simulink model "odziv"  (R2020b)
settings: Solver=ode45  StartTime=0.0  StopTime=Tkon  RelTol=1e-3  EnableMultiTasking=on
libraries: PoKeysIOInterface x1
settings Model: Creator=Administrator  LastModifiedBy=Administrator
settings DataIOCC: LimitDataPoints=on  SaveFormat=Array  ReturnWorkspaceOutputs=off
settings OptimizationCC: LifeSpan=inf
settings DebuggingCC: SolverPrmCheckMsg=warning  SFUnexpectedBacktrackingDiag=warning  SFNoUnconditionalDefaultTransitionDiag=warning  SFExecutionAtInitializationDiag=none  ArithmeticOperatorsInVariantConditions=warning
settings HardwareCC: ProdBitPerPointer=32  ProdBitPerSizeT=32  ProdBitPerPtrDiffT=32  ProdLargestAtomicFloat=None  ProdIntDivRoundTo=Undefined  ProdEndianess=Unspecified  ProdWordSize=32  ProdHWDeviceType=32-bit Generic
settings ModelReferenceCC: PropagateSignalLabelsOutOfModel=off
settings SFSimCC: SimUseLocalCustomCode=off  CustomCodeUndefinedFunction=UseInterfaceOnly
settings RTWCC: RTWUseLocalCustomCode=off
settings CodeAppCC: StateflowObjectComments=on
settings GRTTargetCC: TargetLangStandard=C89/C90 (ANSI)
settings ConfigComp: CovMetricSettings=dw  CovSaveCumulativeToWorkspaceVar=on  CovSaveSingleToWorkspaceVar=on  CovExternalEMLEnable=off  CovSFcnEnable=off

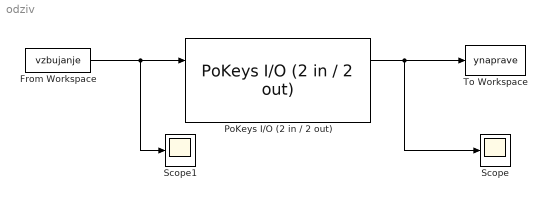
== system odziv ==
  From Workspace : FromWorkspace  VariableName=vzbujanje
  PoKeys I/O (2 in / 2 out) : PoKeysIOInterface/PoKeys I//O (2 in // 2 out)  MaxPowerLimit=100.0  IOTs=0.002  IOSerial=507
      settings: SourceProductName=PoKeys I/O interface
  Scope : Scope
  Scope1 : Scope
  To Workspace : ToWorkspace  VariableName=ynaprave  SaveFormat=Timeseries  SampleTime=-1
  wires:
  PoKeys I/O (2 in / 2 out)/1 -> Scope/1, To Workspace/1
  From Workspace/1 -> PoKeys I/O (2 in / 2 out)/1, Scope1/1
